simulink model "LinLongNormal_Aquila_Claws_Discrete"  (R2017a)
settings: Solver=VariableStepAuto  StartTime=0.0  StopTime=500  RelTol=1e-3  EnableMultiTasking=on
model workspace: external: MAT-File (data not in the file)
undefined symbols (not defined in the file): AP_AltLoop_AltCmdLPFDenTau, AP_AltLoop_altRateCmdMaxLimMps, AP_AltLoop_altRateCmdMinLimMps, AP_AltLoop_Kd, AP_AltLoop_Ki, AP_AltLoop_Ki_WindupMaxLim, AP_AltLoop_Ki_WindupMinLim, AP_AltLoop_Kp, AP_ClimbRate_LPFDenTau, AP_ClimbRateLoop_ClimbRateCmdLPFDenTau, AP_ClimbRateLoop_Ki, AP_ClimbRateLoop_Kp, AP_ClimbRateLoop_LLFiltDenCoe, AP_ClimbRateLoop_LLFiltNumCoe, AP_ClimbRateLoop_MaxPitchCmdrad, AP_ClimbRateLoop_MinPitchCmdrad, AP_FlexLoop_NotchDampingDen, AP_FlexLoop_NotchDampingNum, AP_FlexLoop_NotchFreq, AP_FlexLoop_nzFdbk_Kp, AP_FlexLoop_nzFdbkLLFiltDenCoe, AP_FlexLoop_nzFdbkLLFiltNumCoe, AP_FlexLoop_wn_ElvRollOff, AP_GLALoop_MaxSplCmdDeg, AP_GLALoop_MinSplCmdDeg, AP_GLALoop_nzFdbk_Ki, AP_GLALoop_nzFdbk_Kp, AP_GLALoop_nzFdbkDenTau, AP_GndTrkLoop_CmdLPFDenTau, AP_GndTrkLoop_Kd, AP_GndTrkLoop_Kp, AP_GndTrkLoop_phiCmdMaxLimDeg, AP_GndTrkLoop_phiCmdMinLimDeg, AP_GndTrkLoop_phiRateCmdMaxLimDps, AP_GndTrkLoop_phiRateCmdMinLimDps, AP_PitchLoop_DerivLPFDenTau, AP_PitchLoop_Kd, AP_PitchLoop_Kff, AP_PitchLoop_Ki, AP_PitchLoop_Kp, AP_PitchLoop_Kq, AP_PitchLoop_Notch1BWfactor, AP_PitchLoop_Notch1CosFreqNorm, AP_PitchLoop_qFdbkLFLLFiltDenCoe, AP_PitchLoop_qFdbkLFLLFiltNumCoe, AP_PitchLoop_qFdbkLLFiltDenCoe, AP_PitchLoop_qFdbkLLFiltNumCoe, AP_PitchLoop_thetaCmdLPFDenTau, AP_PitchLoop_wn_ElvRollOff, AP_PitchLoop_zeta_ElvRollOff, AP_PwrLoop_ClimbRateCmdLPFDenTau, AP_PwrLoop_Ki, AP_PwrLoop_Kp, AP_PwrLoop_Kvadv, AP_PwrLoop_LLFiltDenCoe, AP_PwrLoop_LLFiltNumCoe, AP_PwrLoop_MaxThrCmdNorm, AP_PwrLoop_MinThrCmdNorm, AP_PwrLoop_wn_ThrRollOff, AP_PwrLoop_zeta_ThrRollOff ... (+59)
libraries: discretizing x18, aerolibconvert2 x15, simulink x10, Washout x1, cstblocks x1
(part 2 of 2)

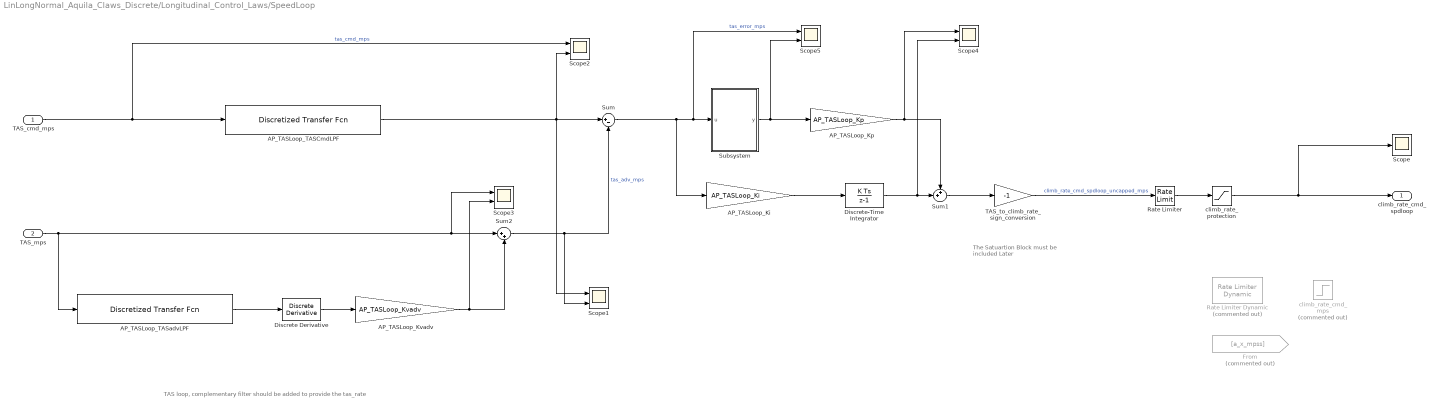
== system LinLongNormal_Aquila_Claws_Discrete/Longitudinal_Control_Laws/SpeedLoop ==
  note: The Satuartion Block must be
      | included Later
  note: TAS loop,
      | complementary filter should be added to provide the tas_rate
  TAS_cmd_mps : Inport
  TAS_mps : Inport  Port=2
  AP_TASLoop_Ki : Gain  Gain=AP_TASLoop_Ki
  AP_TASLoop_Kp : Gain  Gain=AP_TASLoop_Kp
  AP_TASLoop_Kvadv : Gain  Gain=AP_TASLoop_Kvadv
  AP_TASLoop_TASCmdLPF : discretizing/Discretized Transfer Fcn  Numerator=[1]  Denominator=[AP_TASLoop_TASCmdLPFDenTau 1]  AbsTol=auto  SampleTime=Ts  method=zoh  Wc=1
  AP_TASLoop_TASadvLPF : discretizing/Discretized Transfer Fcn  Numerator=[1]  Denominator=[AP_TASLoop_TASadvLPFDenTau 1]  AbsTol=auto  SampleTime=Ts  method=zoh  Wc=1
  Discrete Derivative : simulink/Discrete/Discrete Derivative  gainval=1.0  ICPrevScaledInput=0.0  OutMin=[]  OutMax=[]  OutDataType=fixdt(1, 16)  OutScaling=2^-10  DoSatur=off
  Discrete-Time Integrator : DiscreteIntegrator  InitialConditionSetting=State (most efficient)  SampleTime=-1  ICPrevOutput=DiscIntNeverNeededParam  ICPrevScaledInput=DiscIntNeverNeededParam
  From : From  Commented=on  GotoTag=a_x_mpss  TagVisibility=global
  Rate Limiter : RateLimiter  RisingSlewLimit=AP_TASLoop_ClimbRateCmdRateLimMax  FallingSlewLimit=AP_TASLoop_ClimbRateCmdRateLimMin  SampleTimeMode=inherited
  Rate Limiter Dynamic : simulink/Discontinuities/Rate Limiter Dynamic  Commented=on
      settings: SourceProductName=Simulink
  Scope : Scope
  Scope{1..5} (5 alike) : Scope  NumInputPorts=2
  Subsystem : Subsystem
  Sum : Sum  Inputs=|+-
  Sum1 : Sum  Inputs=++|
  Sum2 : Sum  Inputs=|++
  TAS_to_climb_rate_sign_conversion : Gain  Gain=-1
  climb_rate_cmd_mps : Step  Commented=on  SampleTime=0
  climb_rate_protection : Saturate  UpperLimit=AP_TASLoop_MaxClimbRateCmdmps  LowerLimit=AP_TASLoop_MinClimbRateCmdmps
  climb_rate_cmd_spdloop : Outport
  wires:
  Sum1/1 -> TAS_to_climb_rate_sign_conversion/1
  AP_TASLoop_Ki/1 -> Discrete-Time Integrator/1
  Sum/1 -> AP_TASLoop_Ki/1, Scope5/1, Subsystem/1(u)  "tas_error_mps"
  Discrete-Time Integrator/1 -> Scope4/2, Sum1/2
  TAS_cmd_mps/1 -> AP_TASLoop_TASCmdLPF/1, Scope2/1  "tas_cmd_mps"
  TAS_to_climb_rate_sign_conversion/1 -> Rate Limiter/1  "climb_rate_cmd_spdloop_uncapped_mps"
  TAS_mps/1 -> Scope3/1, Sum2/1, AP_TASLoop_TASadvLPF/1
  AP_TASLoop_TASCmdLPF/1 -> Scope1/1, Scope2/2, Sum/1
  Sum2/1 -> Scope1/2, Sum/2  "tas_adv_mps"
  AP_TASLoop_TASadvLPF/1 -> Discrete Derivative/1
  Discrete Derivative/1 -> AP_TASLoop_Kvadv/1
  AP_TASLoop_Kvadv/1 -> Scope3/2, Sum2/2
  Subsystem/1(y) -> AP_TASLoop_Kp/1, Scope5/2
  AP_TASLoop_Kp/1 -> Scope4/1, Sum1/1
  Rate Limiter/1 -> climb_rate_protection/1
  climb_rate_protection/1 -> climb_rate_cmd_spdloop/1, Scope/1

== system LinLongNormal_Aquila_Claws_Discrete/Lateral_Directional_Control_Laws/GndTrkLoop/pi Bound ==
  In : Inport
  2pi : Constant  Value=2*pi
  Math Function : Math  Operator=mod  SaturateOnIntegerOverflow=on
  Sum1 : Sum  Inputs=|+-  SaturateOnIntegerOverflow=on  InputSameDT=on  OutDataTypeStr=Inherit: Same as first input
  Sum2 : Sum  Inputs=|++  SaturateOnIntegerOverflow=on  InputSameDT=on  OutDataTypeStr=Inherit: Same as first input
  pi : Constant  Value=pi
  Out : Outport
  wires:
  Sum1/1 -> Out/1
  pi/1 -> Sum1/2, Sum2/2
  Sum2/1 -> Math Function/1
  In/1 -> Sum2/1
  2pi/1 -> Math Function/2
  Math Function/1 -> Sum1/1

== system LinLongNormal_Aquila_Claws_Discrete/Lateral_Directional_Control_Laws/RollLoop/Notch Filter 1 ==
  note: One of ways to implement it for the scheduling of the AP_RollLoop_Notch1CosFreqNorm across the flight envelop
  note: 2nd order IIR Notch filter
  u : Inport
  AP_RollLoop_Notch1BWfactor : Gain  Gain=AP_RollLoop_Notch1BWfactor
  AP_RollLoop_Notch1BWfactor1 : Gain  Gain=AP_RollLoop_Notch1BWfactor
  AP_RollLoop_Notch1BWfactor2 : Gain  Gain=AP_RollLoop_Notch1BWfactor
  AP_RollLoop_Notch1CosFreqNorm : Gain  Gain=AP_RollLoop_Notch1CosFreqNorm
  AP_RollLoop_Notch1CosFreqNorm1 : Gain  Gain=AP_RollLoop_Notch1CosFreqNorm
  Delay : Delay  DelayLength=1  InitialCondition=0  SampleTime=Ts
  Delay1 : Delay  DelayLength=1  InitialCondition=0  SampleTime=Ts
  Delay2 : Delay  InitialCondition=0  SampleTime=Ts
  Delay3 : Delay  InitialCondition=0  SampleTime=Ts
  Gain1 : Gain  Gain=-2
  Gain2 : Gain  Gain=0.4697
  Gain4 : Gain  Gain=2
  Gain5 : Gain  Gain=-1
  Sum : Sum  Inputs=|++
  Sum1 : Sum  Inputs=|++
  Sum2 : Sum  Inputs=|++
  Sum3 : Sum  Inputs=+++||
  y : Outport
  wires:
  Sum/1 -> Gain2/1
  AP_RollLoop_Notch1BWfactor/1 -> Sum/1
  AP_RollLoop_Notch1CosFreqNorm/1 -> Sum3/2
  u/1 -> Delay/1, Sum3/1, Delay2/1
  Sum1/1 -> y/1, Delay1/1, Delay3/1
  AP_RollLoop_Notch1BWfactor2/1 -> Gain5/1
  Delay3/1 -> AP_RollLoop_Notch1BWfactor2/1
  Gain1/1 -> AP_RollLoop_Notch1CosFreqNorm/1
  Delay1/1 -> AP_RollLoop_Notch1CosFreqNorm1/1
  Delay2/1 -> Sum3/3
  Delay/1 -> Gain1/1
  AP_RollLoop_Notch1CosFreqNorm1/1 -> Gain4/1
  Sum3/1 -> Sum/2, AP_RollLoop_Notch1BWfactor/1
  Gain2/1 -> Sum1/1
  Gain4/1 -> Sum2/2
  Gain5/1 -> Sum2/1
  AP_RollLoop_Notch1BWfactor1/1 -> Sum1/2
  Sum2/1 -> AP_RollLoop_Notch1BWfactor1/1

== system LinLongNormal_Aquila_Claws_Discrete/Lateral_Directional_Control_Laws/RollLoop/Subsystem1 ==
  u : Inport
  AP_RollLoop_pFdbkLLFiltDenCoe : Gain  Gain=AP_RollLoop_pFdbkLLFiltDenCoe
  AP_RollLoop_pFdbkLLFiltNumCoe : Gain  Gain=AP_RollLoop_pFdbkLLFiltNumCoe
  Delay : Delay  DelayLength=1  InitialCondition=0  SampleTime=Ts
  Delay1 : Delay  DelayLength=1  InitialCondition=0  SampleTime=Ts
  Sum3 : Sum  Inputs=+|+|-
  y : Outport
  wires:
  AP_RollLoop_pFdbkLLFiltDenCoe/1 -> Sum3/3
  u/1 -> AP_RollLoop_pFdbkLLFiltNumCoe/1, Sum3/1
  Delay1/1 -> AP_RollLoop_pFdbkLLFiltDenCoe/1
  AP_RollLoop_pFdbkLLFiltNumCoe/1 -> Delay/1
  Delay/1 -> Sum3/2
  Sum3/1 -> y/1, Delay1/1

== system LinLongNormal_Aquila_Claws_Discrete/Lateral_Directional_Control_Laws/RollLoop/Subsystem2 ==
  u : Inport
  AP_RollLoop_pFdbkLFLLFiltDenCoe : Gain  Gain=AP_RollLoop_pFdbkLFLLFiltDenCoe
  AP_RollLoop_pFdbkLFLLFiltNumCoe : Gain  Gain=AP_RollLoop_pFdbkLFLLFiltNumCoe
  Delay : Delay  DelayLength=1  InitialCondition=0  SampleTime=Ts
  Delay1 : Delay  DelayLength=1  InitialCondition=0  SampleTime=Ts
  Sum3 : Sum  Inputs=+|+|-
  y : Outport
  wires:
  AP_RollLoop_pFdbkLFLLFiltDenCoe/1 -> Sum3/3
  u/1 -> AP_RollLoop_pFdbkLFLLFiltNumCoe/1, Sum3/1
  Delay1/1 -> AP_RollLoop_pFdbkLFLLFiltDenCoe/1
  AP_RollLoop_pFdbkLFLLFiltNumCoe/1 -> Delay/1
  Delay/1 -> Sum3/2
  Sum3/1 -> y/1, Delay1/1

== system LinLongNormal_Aquila_Claws_Discrete/Lateral_Directional_Control_Laws/YawLoop/Subsystem ==
  u : Inport
  AP_YawRateLoop_LLFiltDenCoe : Gain  Gain=AP_YawRateLoop_LLFiltDenCoe
  AP_YawRateLoop_LLFiltNumCoe : Gain  Gain=AP_YawRateLoop_LLFiltNumCoe
  Delay : Delay  DelayLength=1  InitialCondition=0  SampleTime=Ts
  Delay1 : Delay  DelayLength=1  InitialCondition=0  SampleTime=Ts
  Sum3 : Sum  Inputs=+|+|-
  y : Outport
  wires:
  AP_YawRateLoop_LLFiltDenCoe/1 -> Sum3/3
  u/1 -> AP_YawRateLoop_LLFiltNumCoe/1, Sum3/1
  Delay1/1 -> AP_YawRateLoop_LLFiltDenCoe/1
  AP_YawRateLoop_LLFiltNumCoe/1 -> Delay/1
  Delay/1 -> Sum3/2
  Sum3/1 -> y/1, Delay1/1

== system LinLongNormal_Aquila_Claws_Discrete/Longitudinal_Control_Laws/ClimbRateLoop/Subsystem ==
  u : Inport
  AP_ClimbRateLoop_LLFiltDenCoe : Gain  Gain=AP_ClimbRateLoop_LLFiltDenCoe
  AP_ClimbRateLoop_LLFiltNumCoe : Gain  Gain=AP_ClimbRateLoop_LLFiltNumCoe
  Delay : Delay  DelayLength=1  InitialCondition=0  SampleTime=Ts
  Delay1 : Delay  DelayLength=1  InitialCondition=0  SampleTime=Ts
  Sum3 : Sum  Inputs=+|+|-
  y : Outport
  wires:
  AP_ClimbRateLoop_LLFiltDenCoe/1 -> Sum3/3
  u/1 -> AP_ClimbRateLoop_LLFiltNumCoe/1, Sum3/1
  Delay1/1 -> AP_ClimbRateLoop_LLFiltDenCoe/1
  AP_ClimbRateLoop_LLFiltNumCoe/1 -> Delay/1
  Delay/1 -> Sum3/2
  Sum3/1 -> y/1, Delay1/1

== system LinLongNormal_Aquila_Claws_Discrete/Longitudinal_Control_Laws/PitchLoop/Notch Filter 1 ==
  note: One of ways to implement it for the scheduling of the AP_PitchLoop_Notch1CosFreqNorm across the flight envelop
  note: 2nd order IIR Notch filter
  u : Inport
  AP_PitchLoop_Notch1BWfactor : Gain  Gain=AP_PitchLoop_Notch1BWfactor
  AP_PitchLoop_Notch1BWfactor1 : Gain  Gain=AP_PitchLoop_Notch1BWfactor
  AP_PitchLoop_Notch1BWfactor2 : Gain  Gain=AP_PitchLoop_Notch1BWfactor
  AP_PitchLoop_Notch1CosFreqNorm : Gain  Gain=AP_PitchLoop_Notch1CosFreqNorm
  AP_PitchLoop_Notch1CosFreqNorm1 : Gain  Gain=AP_PitchLoop_Notch1CosFreqNorm
  Delay : Delay  DelayLength=1  InitialCondition=0  SampleTime=Ts
  Delay1 : Delay  DelayLength=1  InitialCondition=0  SampleTime=Ts
  Delay2 : Delay  InitialCondition=0  SampleTime=Ts
  Delay3 : Delay  InitialCondition=0  SampleTime=Ts
  Gain1 : Gain  Gain=-2
  Gain2 : Gain  Gain=0.4697
  Gain4 : Gain  Gain=2
  Gain5 : Gain  Gain=-1
  Sum : Sum  Inputs=|++
  Sum1 : Sum  Inputs=|++
  Sum2 : Sum  Inputs=|++
  Sum3 : Sum  Inputs=+++||
  y : Outport
  wires:
  Sum/1 -> Gain2/1
  AP_PitchLoop_Notch1BWfactor/1 -> Sum/1
  AP_PitchLoop_Notch1CosFreqNorm/1 -> Sum3/2
  u/1 -> Delay/1, Sum3/1, Delay2/1
  Sum1/1 -> y/1, Delay1/1, Delay3/1
  AP_PitchLoop_Notch1BWfactor2/1 -> Gain5/1
  Delay3/1 -> AP_PitchLoop_Notch1BWfactor2/1
  Gain1/1 -> AP_PitchLoop_Notch1CosFreqNorm/1
  Delay1/1 -> AP_PitchLoop_Notch1CosFreqNorm1/1
  Delay2/1 -> Sum3/3
  Delay/1 -> Gain1/1
  AP_PitchLoop_Notch1CosFreqNorm1/1 -> Gain4/1
  Sum3/1 -> Sum/2, AP_PitchLoop_Notch1BWfactor/1
  Gain2/1 -> Sum1/1
  Gain4/1 -> Sum2/2
  Gain5/1 -> Sum2/1
  AP_PitchLoop_Notch1BWfactor1/1 -> Sum1/2
  Sum2/1 -> AP_PitchLoop_Notch1BWfactor1/1

== system LinLongNormal_Aquila_Claws_Discrete/Longitudinal_Control_Laws/PitchLoop/Subsystem ==
  u : Inport
  AP_PitchLoop_qFdbkLLFiltDenCoe : Gain  Gain=AP_PitchLoop_qFdbkLLFiltDenCoe
  AP_PitchLoop_qFdbkLLFiltNumCoe : Gain  Gain=AP_PitchLoop_qFdbkLLFiltNumCoe
  Delay : Delay  DelayLength=1  InitialCondition=0  SampleTime=Ts
  Delay1 : Delay  DelayLength=1  InitialCondition=0  SampleTime=Ts
  Sum3 : Sum  Inputs=+|+|-
  y : Outport
  wires:
  AP_PitchLoop_qFdbkLLFiltDenCoe/1 -> Sum3/3
  u/1 -> AP_PitchLoop_qFdbkLLFiltNumCoe/1, Sum3/1
  Delay1/1 -> AP_PitchLoop_qFdbkLLFiltDenCoe/1
  AP_PitchLoop_qFdbkLLFiltNumCoe/1 -> Delay/1
  Delay/1 -> Sum3/2
  Sum3/1 -> y/1, Delay1/1

== system LinLongNormal_Aquila_Claws_Discrete/Longitudinal_Control_Laws/PitchLoop/Subsystem1 ==
  u : Inport
  AP_PitchLoop_qFdbkLFLLFiltDenCoe : Gain  Gain=AP_PitchLoop_qFdbkLFLLFiltDenCoe
  AP_PitchLoop_qFdbkLFLLFiltNumCoe : Gain  Gain=AP_PitchLoop_qFdbkLFLLFiltNumCoe
  Delay : Delay  DelayLength=1  InitialCondition=0  SampleTime=Ts
  Delay1 : Delay  DelayLength=1  InitialCondition=0  SampleTime=Ts
  Sum3 : Sum  Inputs=+|+|-
  y : Outport
  wires:
  AP_PitchLoop_qFdbkLFLLFiltDenCoe/1 -> Sum3/3
  u/1 -> AP_PitchLoop_qFdbkLFLLFiltNumCoe/1, Sum3/1
  Delay1/1 -> AP_PitchLoop_qFdbkLFLLFiltDenCoe/1
  AP_PitchLoop_qFdbkLFLLFiltNumCoe/1 -> Delay/1
  Delay/1 -> Sum3/2
  Sum3/1 -> y/1, Delay1/1

== system LinLongNormal_Aquila_Claws_Discrete/Longitudinal_Control_Laws/PwrLoop/Subsystem ==
  u : Inport
  AP_PwrLoop_LLFiltDenCoe : Gain  Gain=AP_PwrLoop_LLFiltDenCoe
  AP_PwrLoop_LLFiltNumCoe : Gain  Gain=AP_PwrLoop_LLFiltNumCoe
  Delay : Delay  DelayLength=1  InitialCondition=0  SampleTime=Ts
  Delay1 : Delay  DelayLength=1  InitialCondition=0  SampleTime=Ts
  Sum3 : Sum  Inputs=+|+|-
  y : Outport
  wires:
  AP_PwrLoop_LLFiltDenCoe/1 -> Sum3/3
  u/1 -> AP_PwrLoop_LLFiltNumCoe/1, Sum3/1
  Delay1/1 -> AP_PwrLoop_LLFiltDenCoe/1
  AP_PwrLoop_LLFiltNumCoe/1 -> Delay/1
  Delay/1 -> Sum3/2
  Sum3/1 -> y/1, Delay1/1

== system LinLongNormal_Aquila_Claws_Discrete/Longitudinal_Control_Laws/SpeedLoop/Subsystem ==
  u : Inport
  AP_TASLoop_LLFiltDenCoe : Gain  Gain=AP_TASLoop_LLFiltDenCoe
  AP_TASLoop_LLFiltNumCoe : Gain  Gain=AP_TASLoop_LLFiltNumCoe
  Delay : Delay  DelayLength=1  InitialCondition=0  SampleTime=Ts
  Delay1 : Delay  DelayLength=1  InitialCondition=0  SampleTime=Ts
  Sum3 : Sum  Inputs=+|+|-
  y : Outport
  wires:
  AP_TASLoop_LLFiltDenCoe/1 -> Sum3/3
  u/1 -> AP_TASLoop_LLFiltNumCoe/1, Sum3/1
  Delay1/1 -> AP_TASLoop_LLFiltDenCoe/1
  AP_TASLoop_LLFiltNumCoe/1 -> Delay/1
  Delay/1 -> Sum3/2
  Sum3/1 -> y/1, Delay1/1
